simulink model "drone"  (Simulink 6.1)
settings: Solver=ode5  StartTime=0.0  StopTime=90  FixedStep=1e-3  RelTol=1e-3
values from neighbouring files (symbols this model uses):
  Aerodynamique =     [Test en vol.mat]
  Correcteur =     [Test en vol.mat]
  Mecanique =     [Test en vol.mat]
libraries: mblibv1 x43, simulink x26, aerolibtransform2 x4, electricdrivelib x1
(part 2 of 2)

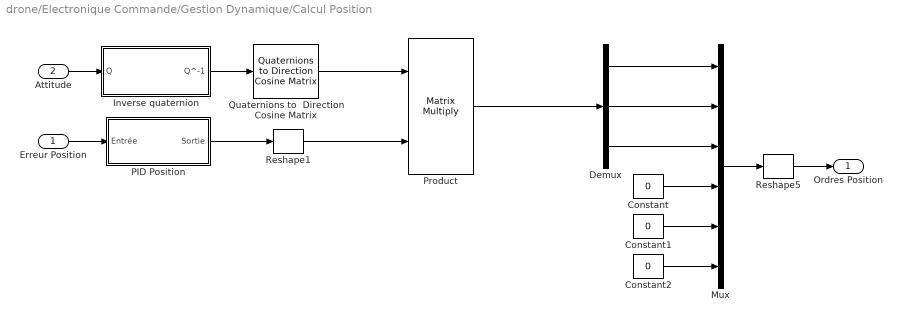
== system drone/Electronique Commande/Gestion Dynamique/Calcul Position ==
  Erreur Position : Inport  Port=1  LatchInput=off
  Attitude : Inport  Port=2  LatchInput=off
  Constant : Constant  Value=0
  Constant1 : Constant  Value=0
  Constant2 : Constant  Value=0
  Demux : Demux  Outputs=3
  Inverse quaternion : Subsystem
  Mux : Mux  Inputs=6
  PID Position : Subsystem
  Product : Product  Multiplication=Matrix(*)  RndMeth=Zero
  Quaternions to  Direction Cosine Matrix : aerolibtransform2/Quaternions to  Direction Cosine Matrix
  Reshape1 : simulink/Math Operations/Reshape  OutputDimensionality=1-D array  OutputDimensions=[1,1]
  Reshape5 : simulink/Math Operations/Reshape  OutputDimensionality=1-D array  OutputDimensions=[1,1]
  Ordres Position : Outport
      settings: BusObject=perturbations
  wires:
  Erreur Position/1 -> PID Position/1(Entrée)
  Mux/1 -> Reshape5/1
  Reshape5/1 -> Ordres Position/1
  Demux/1 -> Mux/1
  Demux/2 -> Mux/2
  Demux/3 -> Mux/3
  Constant2/1 -> Mux/6
  Constant1/1 -> Mux/5
  Constant/1 -> Mux/4
  Attitude/1 -> Inverse quaternion/1(Q)
  Quaternions to  Direction Cosine Matrix/1 -> Product/1
  Reshape1/1 -> Product/2
  Product/1 -> Demux/1
  Inverse quaternion/1(Q^-1) -> Quaternions to  Direction Cosine Matrix/1
  PID Position/1(Sortie) -> Reshape1/1

== system drone/Electronique Commande/Gestion Dynamique/Concatenation composantes ==
  Ordres position : Inport  Port=1  LatchInput=off
  Ordres attitude : Inport  Port=2  LatchInput=off
  Sum : Sum
  Ordres : Outport
      settings: BusObject=perturbations
  wires:
  Ordres attitude/1 -> Sum/2
  Sum/1 -> Ordres/1
  Ordres position/1 -> Sum/1

== system drone/Electronique Commande/Gestion Dynamique/Extraction attitude ==
  Etat : Inport  Port=1  LatchInput=off
  Demux1 : Demux  Outputs=7
  Mux : Mux  Inputs=3
  Mux1 : Mux
  Reshape : simulink/Math Operations/Reshape  OutputDimensionality=1-D array  OutputDimensions=[1,1]
  Terminator : Terminator
  Attitude : Outport
      settings: BusObject=perturbations
  wires:
  Etat/1 -> Demux1/1
  Demux1/4 -> Mux1/1
  Demux1/5 -> Mux1/2
  Demux1/6 -> Mux1/3
  Demux1/7 -> Mux1/4
  Demux1/3 -> Mux/3
  Demux1/2 -> Mux/2
  Demux1/1 -> Mux/1
  Mux1/1 -> Reshape/1
  Mux/1 -> Terminator/1
  Reshape/1 -> Attitude/1

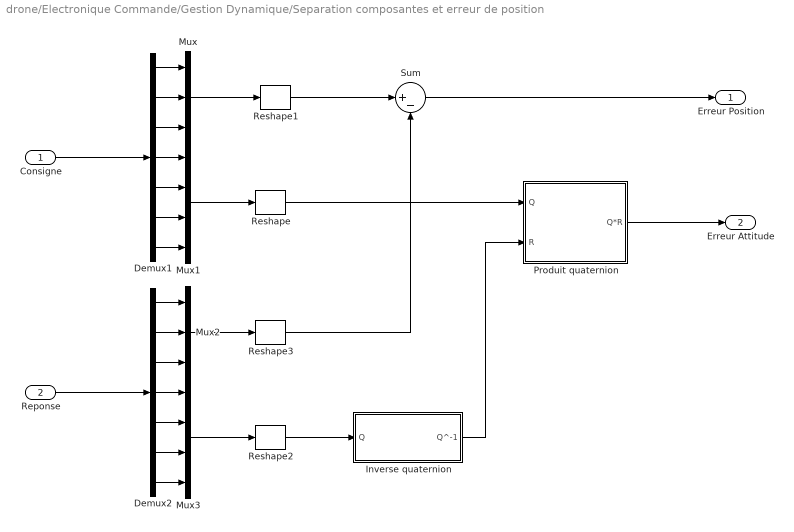
== system drone/Electronique Commande/Gestion Dynamique/Separation composantes et erreur de position ==
  Consigne : Inport  Port=1  LatchInput=off
  Reponse : Inport  Port=2  LatchInput=off
  Demux1 : Demux  Outputs=7
  Demux2 : Demux  Outputs=7
  Inverse quaternion : Subsystem
  Mux : Mux  Inputs=3
  Mux1 : Mux
  Mux2 : Mux  Inputs=3
  Mux3 : Mux
  Produit quaternion : Subsystem
  Reshape{,1..3} (4 alike) : simulink/Math Operations/Reshape  OutputDimensionality=1-D array  OutputDimensions=[1,1]
  Sum : Sum  Inputs=|+-
  Erreur Position : Outport
      settings: BusObject=perturbations
  Erreur Attitude : Outport  Port=2
      settings: BusObject=perturbations
  wires:
  Consigne/1 -> Demux1/1
  Demux1/4 -> Mux1/1
  Demux1/5 -> Mux1/2
  Demux1/6 -> Mux1/3
  Demux1/7 -> Mux1/4
  Demux1/3 -> Mux/3
  Demux1/2 -> Mux/2
  Demux1/1 -> Mux/1
  Mux1/1 -> Reshape/1
  Mux/1 -> Reshape1/1
  Demux2/4 -> Mux3/1
  Demux2/5 -> Mux3/2
  Demux2/6 -> Mux3/3
  Demux2/7 -> Mux3/4
  Demux2/3 -> Mux2/3
  Demux2/2 -> Mux2/2
  Demux2/1 -> Mux2/1
  Reponse/1 -> Demux2/1
  Mux3/1 -> Reshape2/1
  Mux2/1 -> Reshape3/1
  Reshape1/1 -> Sum/1
  Reshape3/1 -> Sum/2
  Sum/1 -> Erreur Position/1
  Reshape2/1 -> Inverse quaternion/1(Q)
  Reshape/1 -> Produit quaternion/1(Q)
  Inverse quaternion/1(Q^-1) -> Produit quaternion/2(R)
  Produit quaternion/1(Q*R) -> Erreur Attitude/1

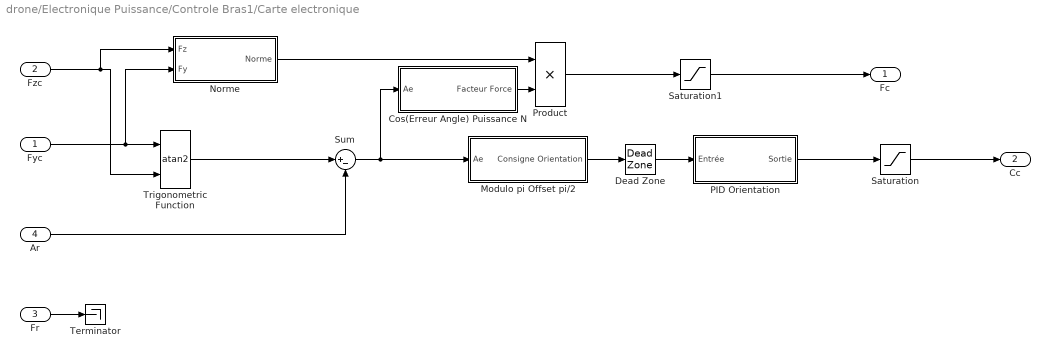
== system drone/Electronique Puissance/Controle Bras1/Carte electronique ==
  Fyc : Inport  Port=1  LatchInput=off
  Fzc : Inport  Port=2  LatchInput=off
  Fr : Inport  Port=3  LatchInput=off
  Ar : Inport  Port=4  LatchInput=off
  Cos(Erreur Angle) Puissance N : Subsystem
  Dead Zone : DeadZone  LowerValue=-Correcteur.Orientation.DZ  UpperValue=Correcteur.Orientation.DZ  SaturateOnIntegerOverflow=on
  Modulo pi Offset pi/2 : Subsystem
  Norme : Subsystem
  PID Orientation : Subsystem
  Product : Product  RndMeth=Zero
  Saturation : Saturate  UpperLimit=Mecanique.Bras.Csat  LowerLimit=-Mecanique.Bras.Csat
  Saturation1 : Saturate  UpperLimit=Mecanique.Rotor.Fsat  LowerLimit=-Mecanique.Rotor.Fsat
  Sum : Sum  Inputs=|+-
  Terminator : Terminator
  Trigonometric Function : Trigonometry  Operator=atan2  OutputSignalType=real
  Fc : Outport
  Cc : Outport  Port=2
  wires:
  Fzc/1 -> Trigonometric Function/2, Norme/1(Fz)
  Fyc/1 -> Trigonometric Function/1, Norme/2(Fy)
  Trigonometric Function/1 -> Sum/1
  Norme/1(Norme) -> Product/1
  Ar/1 -> Sum/2
  Sum/1 -> Modulo pi Offset pi/2/1(Ae), Cos(Erreur Angle) Puissance N/1(Ae)
  Fr/1 -> Terminator/1
  Cos(Erreur Angle) Puissance N/1(Facteur Force) -> Product/2
  Product/1 -> Saturation1/1
  Modulo pi Offset pi/2/1(Consigne Orientation) -> Dead Zone/1
  Saturation/1 -> Cc/1
  PID Orientation/1(Sortie) -> Saturation/1
  Saturation1/1 -> Fc/1
  Dead Zone/1 -> PID Orientation/1(Entrée)

== system drone/Electronique Puissance/Controle Bras1/Moteur orientation ==
  Fz : Inport  Port=1  LatchInput=off
  Couple : Outport

== system drone/Electronique Puissance/Controle Bras1/Moteur propulsion ==
  Fz : Inport  Port=1  LatchInput=off
  Couple : Outport

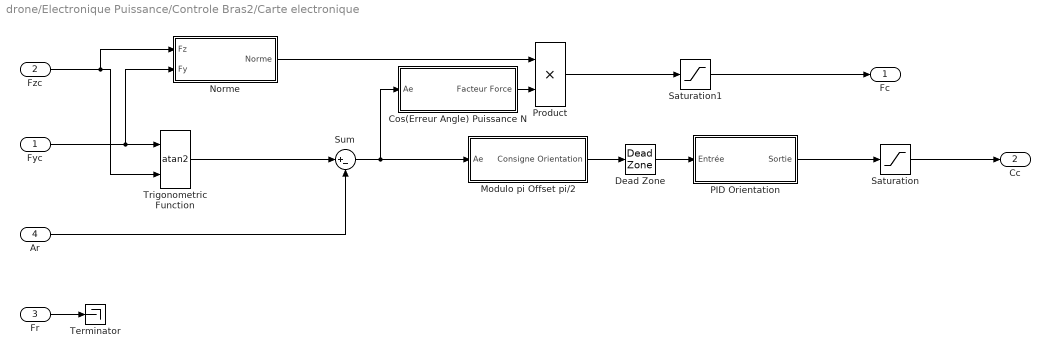
== system drone/Electronique Puissance/Controle Bras2/Carte electronique ==
  Fyc : Inport  Port=1  LatchInput=off
  Fzc : Inport  Port=2  LatchInput=off
  Fr : Inport  Port=3  LatchInput=off
  Ar : Inport  Port=4  LatchInput=off
  Cos(Erreur Angle) Puissance N : Subsystem
  Dead Zone : DeadZone  LowerValue=-Correcteur.Orientation.DZ  UpperValue=Correcteur.Orientation.DZ  SaturateOnIntegerOverflow=on
  Modulo pi Offset pi/2 : Subsystem
  Norme : Subsystem
  PID Orientation : Subsystem
  Product : Product  RndMeth=Zero
  Saturation : Saturate  UpperLimit=Mecanique.Bras.Csat  LowerLimit=-Mecanique.Bras.Csat
  Saturation1 : Saturate  UpperLimit=Mecanique.Rotor.Fsat  LowerLimit=-Mecanique.Rotor.Fsat
  Sum : Sum  Inputs=|+-
  Terminator : Terminator
  Trigonometric Function : Trigonometry  Operator=atan2  OutputSignalType=real
  Fc : Outport
  Cc : Outport  Port=2
  wires:
  Fzc/1 -> Trigonometric Function/2, Norme/1(Fz)
  Fyc/1 -> Trigonometric Function/1, Norme/2(Fy)
  Trigonometric Function/1 -> Sum/1
  Norme/1(Norme) -> Product/1
  Ar/1 -> Sum/2
  Sum/1 -> Modulo pi Offset pi/2/1(Ae), Cos(Erreur Angle) Puissance N/1(Ae)
  Fr/1 -> Terminator/1
  Cos(Erreur Angle) Puissance N/1(Facteur Force) -> Product/2
  Product/1 -> Saturation1/1
  Modulo pi Offset pi/2/1(Consigne Orientation) -> Dead Zone/1
  Saturation/1 -> Cc/1
  PID Orientation/1(Sortie) -> Saturation/1
  Saturation1/1 -> Fc/1
  Dead Zone/1 -> PID Orientation/1(Entrée)

== system drone/Electronique Puissance/Controle Bras2/Moteur orientation ==
  Fz : Inport  Port=1  LatchInput=off
  Couple : Outport

== system drone/Electronique Puissance/Controle Bras2/Moteur propulsion ==
  Fz : Inport  Port=1  LatchInput=off
  Couple : Outport

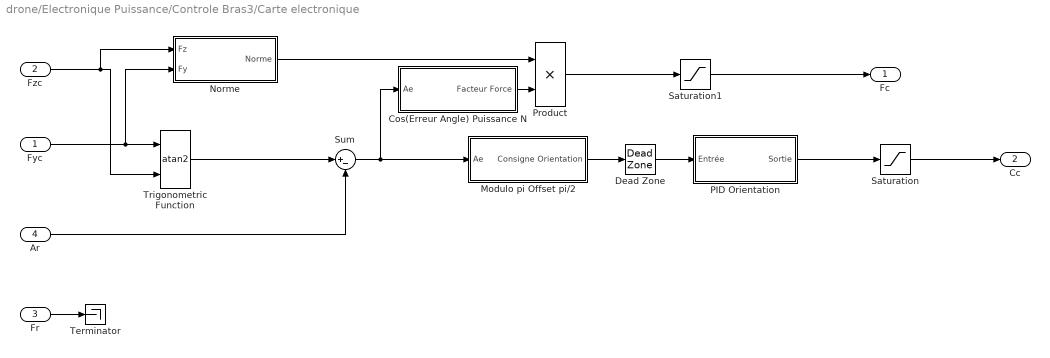
== system drone/Electronique Puissance/Controle Bras3/Carte electronique ==
  Fyc : Inport  Port=1  LatchInput=off
  Fzc : Inport  Port=2  LatchInput=off
  Fr : Inport  Port=3  LatchInput=off
  Ar : Inport  Port=4  LatchInput=off
  Cos(Erreur Angle) Puissance N : Subsystem
  Dead Zone : DeadZone  LowerValue=-Correcteur.Orientation.DZ  UpperValue=Correcteur.Orientation.DZ  SaturateOnIntegerOverflow=on
  Modulo pi Offset pi/2 : Subsystem
  Norme : Subsystem
  PID Orientation : Subsystem
  Product : Product  RndMeth=Zero
  Saturation : Saturate  UpperLimit=Mecanique.Bras.Csat  LowerLimit=-Mecanique.Bras.Csat
  Saturation1 : Saturate  UpperLimit=Mecanique.Rotor.Fsat  LowerLimit=-Mecanique.Rotor.Fsat
  Sum : Sum  Inputs=|+-
  Terminator : Terminator
  Trigonometric Function : Trigonometry  Operator=atan2  OutputSignalType=real
  Fc : Outport
  Cc : Outport  Port=2
  wires:
  Fzc/1 -> Trigonometric Function/2, Norme/1(Fz)
  Fyc/1 -> Trigonometric Function/1, Norme/2(Fy)
  Trigonometric Function/1 -> Sum/1
  Norme/1(Norme) -> Product/1
  Ar/1 -> Sum/2
  Sum/1 -> Modulo pi Offset pi/2/1(Ae), Cos(Erreur Angle) Puissance N/1(Ae)
  Fr/1 -> Terminator/1
  Cos(Erreur Angle) Puissance N/1(Facteur Force) -> Product/2
  Product/1 -> Saturation1/1
  Modulo pi Offset pi/2/1(Consigne Orientation) -> Dead Zone/1
  Saturation/1 -> Cc/1
  PID Orientation/1(Sortie) -> Saturation/1
  Saturation1/1 -> Fc/1
  Dead Zone/1 -> PID Orientation/1(Entrée)

== system drone/Electronique Puissance/Controle Bras3/Moteur orientation ==
  Fz : Inport  Port=1  LatchInput=off
  Couple : Outport

== system drone/Electronique Puissance/Controle Bras3/Moteur propulsion ==
  Fz : Inport  Port=1  LatchInput=off
  Couple : Outport

== system drone/Electronique Commande/Gestion Dynamique/Calcul Attitude/Inverse quaternion ==
  Q : Inport  Port=1  LatchInput=off
  Gain : Gain  Gain=[1 -1 -1 -1]
  Q^-1 : Outport
  wires:
  Q/1 -> Gain/1
  Gain/1 -> Q^-1/1

== system drone/Electronique Commande/Gestion Dynamique/Calcul Attitude/Norme ==
  Entrée : Inport  Port=1  LatchInput=off
  Add : Sum  Inputs=+++  OutScaling=2^-10
  Carré : simulink/Math Operations/Polynomial  coefs=[1 0 0]
  Carré1 : simulink/Math Operations/Polynomial  coefs=[1 0 0]
  Carré2 : simulink/Math Operations/Polynomial  coefs=[1 0 0]
  Demux2 : Demux  Outputs=3
  Math Function : Math  Operator=sqrt  SaturateOnIntegerOverflow=on
  Sortie : Outport
      settings: BusObject=perturbations
  wires:
  Math Function/1 -> Sortie/1
  Carré/1 -> Add/1
  Add/1 -> Math Function/1
  Carré1/1 -> Add/2
  Carré2/1 -> Add/3
  Demux2/2 -> Carré1/1
  Demux2/1 -> Carré/1
  Demux2/3 -> Carré2/1
  Entrée/1 -> Demux2/1

== system drone/Electronique Commande/Gestion Dynamique/Calcul Attitude/Norme1 ==
  Entrée : Inport  Port=1  LatchInput=off
  Add : Sum  Inputs=+++  OutScaling=2^-10
  Carré : simulink/Math Operations/Polynomial  coefs=[1 0 0]
  Carré1 : simulink/Math Operations/Polynomial  coefs=[1 0 0]
  Carré2 : simulink/Math Operations/Polynomial  coefs=[1 0 0]
  Demux2 : Demux  Outputs=3
  Math Function : Math  Operator=sqrt  SaturateOnIntegerOverflow=on
  Sortie : Outport
      settings: BusObject=perturbations
  wires:
  Math Function/1 -> Sortie/1
  Carré/1 -> Add/1
  Add/1 -> Math Function/1
  Carré1/1 -> Add/2
  Carré2/1 -> Add/3
  Demux2/2 -> Carré1/1
  Demux2/1 -> Carré/1
  Demux2/3 -> Carré2/1
  Entrée/1 -> Demux2/1

== system drone/Electronique Commande/Gestion Dynamique/Calcul Attitude/PID Attitude Ang ==
  Entrée : Inport  Port=1  LatchInput=off
  Derivative : Derivative
  Derivative2 : Derivative
  Gain : Gain  Gain=Correcteur.Attitude.Angle.Kp
  Gain1 : Gain  Gain=Correcteur.Attitude.Angle.Kd
  Gain2 : Gain  Gain=Correcteur.Attitude.Angle.Ki
  Gain3 : Gain  Gain=Correcteur.Attitude.Angle.Kdd
  Integrator : Integrator
  Reshape : simulink/Math Operations/Reshape  OutputDimensionality=1-D array  OutputDimensions=[1,1]
  Sum : Sum  Inputs=++++
  Sortie : Outport
      settings: BusObject=perturbations
  wires:
  Entrée/1 -> Gain/1
  Gain/1 -> Gain1/1, Gain2/1, Sum/3
  Gain2/1 -> Integrator/1
  Gain1/1 -> Derivative/1
  Sum/1 -> Reshape/1
  Reshape/1 -> Sortie/1
  Gain3/1 -> Derivative2/1
  Derivative2/1 -> Sum/1
  Integrator/1 -> Sum/4
  Derivative/1 -> Sum/2, Gain3/1

== system drone/Electronique Commande/Gestion Dynamique/Calcul Attitude/PID Attitude Quat ==
  Entrée : Inport  Port=1  LatchInput=off
  Derivative : Derivative
  Derivative2 : Derivative
  Gain : Gain  Gain=Correcteur.Attitude.Quaternion.Kp
  Gain1 : Gain  Gain=Correcteur.Attitude.Quaternion.Kd
  Gain2 : Gain  Gain=Correcteur.Attitude.Quaternion.Ki
  Gain3 : Gain  Gain=Correcteur.Attitude.Quaternion.Kdd
  Integrator : Integrator
  Reshape : simulink/Math Operations/Reshape  OutputDimensionality=1-D array  OutputDimensions=[1,1]
  Sum : Sum  Inputs=++++
  Sortie : Outport
      settings: BusObject=perturbations
  wires:
  Entrée/1 -> Gain/1
  Gain/1 -> Gain1/1, Gain2/1, Sum/3
  Gain2/1 -> Integrator/1
  Gain1/1 -> Derivative/1
  Sum/1 -> Reshape/1
  Reshape/1 -> Sortie/1
  Gain3/1 -> Derivative2/1
  Derivative2/1 -> Sum/1
  Integrator/1 -> Sum/4
  Derivative/1 -> Sum/2, Gain3/1

== system drone/Electronique Commande/Gestion Dynamique/Calcul Attitude/PID Attitude Vec ==
  Entrée : Inport  Port=1  LatchInput=off
  Derivative : Derivative
  Derivative2 : Derivative
  Gain : Gain  Gain=Correcteur.Attitude.Vecteur.Kp
  Gain1 : Gain  Gain=Correcteur.Attitude.Vecteur.Kd
  Gain2 : Gain  Gain=Correcteur.Attitude.Vecteur.Ki
  Gain3 : Gain  Gain=Correcteur.Attitude.Vecteur.Kdd
  Integrator : Integrator
  Reshape : simulink/Math Operations/Reshape  OutputDimensionality=1-D array  OutputDimensions=[1,1]
  Sum : Sum  Inputs=++++
  Sortie : Outport
      settings: BusObject=perturbations
  wires:
  Entrée/1 -> Gain/1
  Gain/1 -> Gain1/1, Gain2/1, Sum/3
  Gain2/1 -> Integrator/1
  Gain1/1 -> Derivative/1
  Sum/1 -> Reshape/1
  Reshape/1 -> Sortie/1
  Gain3/1 -> Derivative2/1
  Derivative2/1 -> Sum/1
  Integrator/1 -> Sum/4
  Derivative/1 -> Sum/2, Gain3/1

== system drone/Electronique Commande/Gestion Dynamique/Calcul Attitude/inversion non infinie ==
  Entree : Inport  Port=1  LatchInput=off
  Constant : Constant
  Divide : Product  Inputs=/  OutScaling=2^-10
  Switch : Switch  Criteria=u2 > Threshold  ZeroCross=off
  Sortie : Outport
  wires:
  Switch/1 -> Divide/1
  Entree/1 -> Switch/1, Switch/2
  Constant/1 -> Switch/3
  Divide/1 -> Sortie/1

== system drone/Electronique Commande/Gestion Dynamique/Calcul Position/Inverse quaternion ==
  Q : Inport  Port=1  LatchInput=off
  Gain : Gain  Gain=[1 -1 -1 -1]
  Q^-1 : Outport
  wires:
  Q/1 -> Gain/1
  Gain/1 -> Q^-1/1

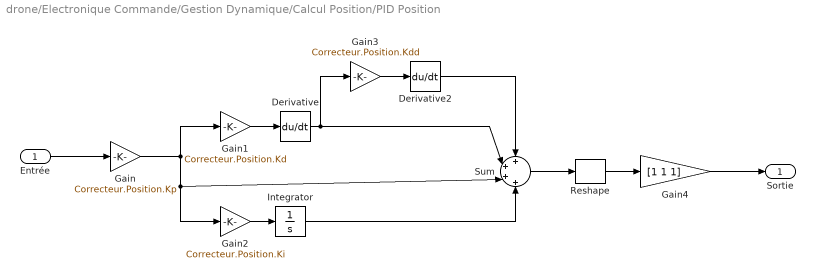
== system drone/Electronique Commande/Gestion Dynamique/Calcul Position/PID Position ==
  Entrée : Inport  Port=1  LatchInput=off
  Derivative : Derivative
  Derivative2 : Derivative
  Gain : Gain  Gain=Correcteur.Position.Kp
  Gain1 : Gain  Gain=Correcteur.Position.Kd
  Gain2 : Gain  Gain=Correcteur.Position.Ki
  Gain3 : Gain  Gain=Correcteur.Position.Kdd
  Gain4 : Gain  Gain=[1 1 1]
  Integrator : Integrator
  Reshape : simulink/Math Operations/Reshape  OutputDimensionality=1-D array  OutputDimensions=[1,1]
  Sum : Sum  Inputs=++++
  Sortie : Outport
      settings: BusObject=perturbations
  wires:
  Entrée/1 -> Gain/1
  Gain/1 -> Gain1/1, Gain2/1, Sum/3
  Gain2/1 -> Integrator/1
  Gain1/1 -> Derivative/1
  Sum/1 -> Reshape/1
  Reshape/1 -> Gain4/1
  Gain3/1 -> Derivative2/1
  Derivative2/1 -> Sum/1
  Integrator/1 -> Sum/4
  Derivative/1 -> Sum/2, Gain3/1
  Gain4/1 -> Sortie/1

== system drone/Electronique Commande/Gestion Dynamique/Separation composantes et erreur de position/Inverse quaternion ==
  Q : Inport  Port=1  LatchInput=off
  Gain : Gain  Gain=[1 -1 -1 -1]
  Q^-1 : Outport
  wires:
  Q/1 -> Gain/1
  Gain/1 -> Q^-1/1

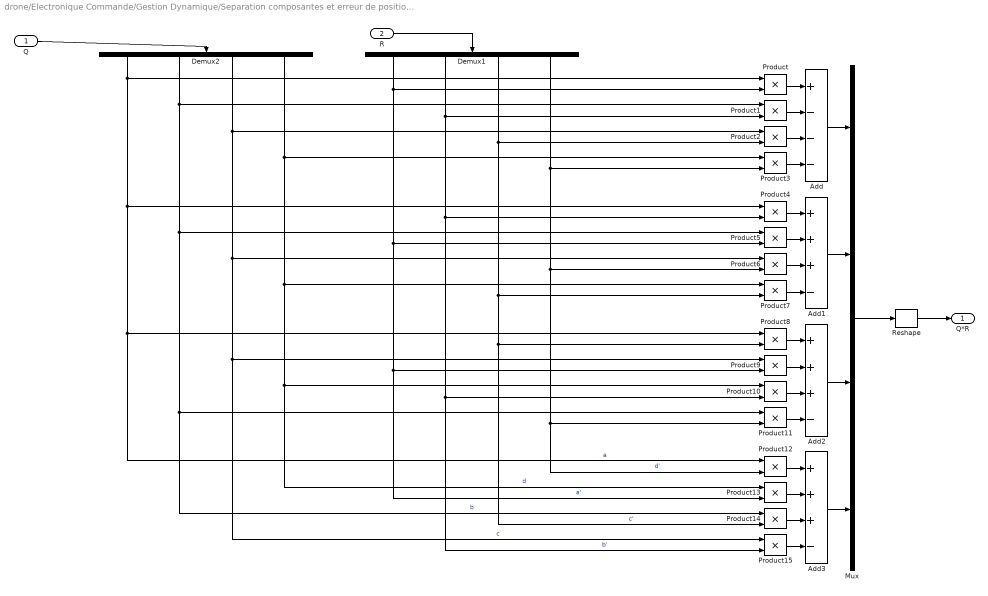
== system drone/Electronique Commande/Gestion Dynamique/Separation composantes et erreur de position/Produit quaternion ==
  Q : Inport  Port=1  LatchInput=off
  R : Inport  Port=2  LatchInput=off
  Add : Sum  Inputs=+---  OutScaling=2^-10
  Add1 : Sum  Inputs=+++-  OutScaling=2^-10
  Add2 : Sum  Inputs=+++-  OutScaling=2^-10
  Add3 : Sum  Inputs=+++-  OutScaling=2^-10
  Demux1 : Demux  Orientation=down
  Demux2 : Demux  Orientation=down
  Mux : Mux
  Product{,1..15} (16 alike) : Product  RndMeth=Zero
  Reshape : simulink/Math Operations/Reshape  OutputDimensionality=1-D array  OutputDimensions=[1,1]
  Q*R : Outport
  wires:
  R/1 -> Demux1/1
  Q/1 -> Demux2/1
  Mux/1 -> Reshape/1
  Reshape/1 -> Q*R/1
  Demux2/1 -> Product/1, Product4/1, Product8/1, Product12/1  "a"
  Add/1 -> Mux/1
  Add1/1 -> Mux/2
  Add2/1 -> Mux/3
  Add3/1 -> Mux/4
  Product3/1 -> Add/4
  Product2/1 -> Add/3
  Product1/1 -> Add/2
  Product/1 -> Add/1
  Product7/1 -> Add1/4
  Product6/1 -> Add1/3
  Product5/1 -> Add1/2
  Product4/1 -> Add1/1
  Product11/1 -> Add2/4
  Product10/1 -> Add2/3
  Product9/1 -> Add2/2
  Product8/1 -> Add2/1
  Product15/1 -> Add3/4
  Product14/1 -> Add3/3
  Product13/1 -> Add3/2
  Product12/1 -> Add3/1
  Demux2/2 -> Product1/1, Product5/1, Product11/1, Product14/1  "b"
  Demux2/3 -> Product2/1, Product6/1, Product9/1, Product15/1  "c"
  Demux2/4 -> Product3/1, Product7/1, Product10/1, Product13/1  "d"
  Demux1/1 -> Product/2, Product5/2, Product9/2, Product13/2  "a'"
  Demux1/2 -> Product1/2, Product4/2, Product10/2, Product15/2  "b'"
  Demux1/3 -> Product2/2, Product7/2, Product8/2, Product14/2  "c'"
  Demux1/4 -> Product3/2, Product6/2, Product11/2, Product12/2  "d'"

== system drone/Electronique Puissance/Controle Bras1/Carte electronique/Cos(Erreur Angle) Puissance N ==
  Ae : Inport  Port=1  LatchInput=off
  Constant : Constant  Value=(Correcteur.Rotor.ExposantFacteurAngulaire*2)+1
  Cos(Erreur  Angle) : Trigonometry  Operator=cos
  Math Function : Math  Operator=pow  SaturateOnIntegerOverflow=on
  Facteur Force : Outport
  wires:
  Ae/1 -> Cos(Erreur  Angle)/1
  Cos(Erreur  Angle)/1 -> Math Function/1
  Constant/1 -> Math Function/2
  Math Function/1 -> Facteur Force/1

== system drone/Electronique Puissance/Controle Bras1/Carte electronique/Modulo pi Offset pi/2 ==
  Ae : Inport  Port=1  LatchInput=off
  Constant : Constant  Value=pi
  Constant1 : Constant  Value=pi/2
  Constant2 : Constant  Value=pi/2
  Math Function : Math  Operator=mod  SaturateOnIntegerOverflow=on
  Sum : Sum  Inputs=|++
  Sum1 : Sum  Inputs=|+-
  Consigne Orientation : Outport
  wires:
  Constant/1 -> Math Function/2
  Sum/1 -> Math Function/1
  Constant1/1 -> Sum/2
  Ae/1 -> Sum/1
  Constant2/1 -> Sum1/2
  Math Function/1 -> Sum1/1
  Sum1/1 -> Consigne Orientation/1

== system drone/Electronique Puissance/Controle Bras1/Carte electronique/Norme ==
  Fz : Inport  Port=1  LatchInput=off
  Fy : Inport  Port=2  LatchInput=off
  Add : Sum  OutScaling=2^-10
  Math Function : Math  Operator=square  SaturateOnIntegerOverflow=on
  Math Function1 : Math  Operator=square  SaturateOnIntegerOverflow=on
  Math Function2 : Math  Operator=sqrt  SaturateOnIntegerOverflow=on
  Norme : Outport
  wires:
  Add/1 -> Math Function2/1
  Math Function1/1 -> Add/1
  Math Function/1 -> Add/2
  Fz/1 -> Math Function1/1
  Fy/1 -> Math Function/1
  Math Function2/1 -> Norme/1

== system drone/Electronique Puissance/Controle Bras1/Carte electronique/PID Orientation ==
  Entrée : Inport  Port=1  LatchInput=off
  Derivative : Derivative
  Gain : Gain  Gain=Correcteur.Orientation.Kp
  Gain1 : Gain  Gain=Correcteur.Orientation.Kd
  Gain2 : Gain  Gain=Correcteur.Orientation.Ki
  Integrator : Integrator
  Sum : Sum  Inputs=+++
  Sortie : Outport
      settings: BusObject=perturbations
  wires:
  Entrée/1 -> Gain/1
  Gain/1 -> Sum/2, Gain1/1, Gain2/1
  Derivative/1 -> Sum/1
  Integrator/1 -> Sum/3
  Gain2/1 -> Integrator/1
  Gain1/1 -> Derivative/1
  Sum/1 -> Sortie/1

== system drone/Electronique Puissance/Controle Bras2/Carte electronique/Cos(Erreur Angle) Puissance N ==
  Ae : Inport  Port=1  LatchInput=off
  Constant : Constant  Value=(Correcteur.Rotor.ExposantFacteurAngulaire*2)+1
  Cos(Erreur  Angle) : Trigonometry  Operator=cos
  Math Function : Math  Operator=pow  SaturateOnIntegerOverflow=on
  Facteur Force : Outport
  wires:
  Ae/1 -> Cos(Erreur  Angle)/1
  Cos(Erreur  Angle)/1 -> Math Function/1
  Constant/1 -> Math Function/2
  Math Function/1 -> Facteur Force/1

== system drone/Electronique Puissance/Controle Bras2/Carte electronique/Modulo pi Offset pi/2 ==
  Ae : Inport  Port=1  LatchInput=off
  Constant : Constant  Value=pi
  Constant1 : Constant  Value=pi/2
  Constant2 : Constant  Value=pi/2
  Math Function : Math  Operator=mod  SaturateOnIntegerOverflow=on
  Sum : Sum  Inputs=|++
  Sum1 : Sum  Inputs=|+-
  Consigne Orientation : Outport
  wires:
  Constant/1 -> Math Function/2
  Sum/1 -> Math Function/1
  Constant1/1 -> Sum/2
  Ae/1 -> Sum/1
  Constant2/1 -> Sum1/2
  Math Function/1 -> Sum1/1
  Sum1/1 -> Consigne Orientation/1

== system drone/Electronique Puissance/Controle Bras2/Carte electronique/Norme ==
  Fz : Inport  Port=1  LatchInput=off
  Fy : Inport  Port=2  LatchInput=off
  Add : Sum  OutScaling=2^-10
  Math Function : Math  Operator=square  SaturateOnIntegerOverflow=on
  Math Function1 : Math  Operator=square  SaturateOnIntegerOverflow=on
  Math Function2 : Math  Operator=sqrt  SaturateOnIntegerOverflow=on
  Norme : Outport
  wires:
  Add/1 -> Math Function2/1
  Math Function1/1 -> Add/1
  Math Function/1 -> Add/2
  Fz/1 -> Math Function1/1
  Fy/1 -> Math Function/1
  Math Function2/1 -> Norme/1

== system drone/Electronique Puissance/Controle Bras2/Carte electronique/PID Orientation ==
  Entrée : Inport  Port=1  LatchInput=off
  Derivative : Derivative
  Gain : Gain  Gain=Correcteur.Orientation.Kp
  Gain1 : Gain  Gain=Correcteur.Orientation.Kd
  Gain2 : Gain  Gain=Correcteur.Orientation.Ki
  Integrator : Integrator
  Sum : Sum  Inputs=+++
  Sortie : Outport
      settings: BusObject=perturbations
  wires:
  Entrée/1 -> Gain/1
  Gain/1 -> Sum/2, Gain1/1, Gain2/1
  Derivative/1 -> Sum/1
  Integrator/1 -> Sum/3
  Gain2/1 -> Integrator/1
  Gain1/1 -> Derivative/1
  Sum/1 -> Sortie/1

== system drone/Electronique Puissance/Controle Bras3/Carte electronique/Cos(Erreur Angle) Puissance N ==
  Ae : Inport  Port=1  LatchInput=off
  Constant : Constant  Value=(Correcteur.Rotor.ExposantFacteurAngulaire*2)+1
  Cos(Erreur  Angle) : Trigonometry  Operator=cos
  Math Function : Math  Operator=pow  SaturateOnIntegerOverflow=on
  Facteur Force : Outport
  wires:
  Ae/1 -> Cos(Erreur  Angle)/1
  Cos(Erreur  Angle)/1 -> Math Function/1
  Constant/1 -> Math Function/2
  Math Function/1 -> Facteur Force/1

== system drone/Electronique Puissance/Controle Bras3/Carte electronique/Modulo pi Offset pi/2 ==
  Ae : Inport  Port=1  LatchInput=off
  Constant : Constant  Value=pi
  Constant1 : Constant  Value=pi/2
  Constant2 : Constant  Value=pi/2
  Math Function : Math  Operator=mod  SaturateOnIntegerOverflow=on
  Sum : Sum  Inputs=|++
  Sum1 : Sum  Inputs=|+-
  Consigne Orientation : Outport
  wires:
  Constant/1 -> Math Function/2
  Sum/1 -> Math Function/1
  Constant1/1 -> Sum/2
  Ae/1 -> Sum/1
  Constant2/1 -> Sum1/2
  Math Function/1 -> Sum1/1
  Sum1/1 -> Consigne Orientation/1

== system drone/Electronique Puissance/Controle Bras3/Carte electronique/Norme ==
  Fz : Inport  Port=1  LatchInput=off
  Fy : Inport  Port=2  LatchInput=off
  Add : Sum  OutScaling=2^-10
  Math Function : Math  Operator=square  SaturateOnIntegerOverflow=on
  Math Function1 : Math  Operator=square  SaturateOnIntegerOverflow=on
  Math Function2 : Math  Operator=sqrt  SaturateOnIntegerOverflow=on
  Norme : Outport
  wires:
  Add/1 -> Math Function2/1
  Math Function1/1 -> Add/1
  Math Function/1 -> Add/2
  Fz/1 -> Math Function1/1
  Fy/1 -> Math Function/1
  Math Function2/1 -> Norme/1

== system drone/Electronique Puissance/Controle Bras3/Carte electronique/PID Orientation ==
  Entrée : Inport  Port=1  LatchInput=off
  Derivative : Derivative
  Gain : Gain  Gain=Correcteur.Orientation.Kp
  Gain1 : Gain  Gain=Correcteur.Orientation.Kd
  Gain2 : Gain  Gain=Correcteur.Orientation.Ki
  Integrator : Integrator
  Sum : Sum  Inputs=+++
  Sortie : Outport
      settings: BusObject=perturbations
  wires:
  Entrée/1 -> Gain/1
  Gain/1 -> Sum/2, Gain1/1, Gain2/1
  Derivative/1 -> Sum/1
  Integrator/1 -> Sum/3
  Gain2/1 -> Integrator/1
  Gain1/1 -> Derivative/1
  Sum/1 -> Sortie/1
